simulink model "identyfikacja_zawor3_reczny"  (R2014b)
settings: Solver=ode5  StartTime=0.0  StopTime=41.25  FixedStep=0.05  RelTol=1e-3
values from neighbouring files (symbols this model uses):
  C3 = q/sqrt(H3pp)    [linearyzacja_analitycznie.m]    (also in wskaznikZawor3.m = parametry(1))
  R = 40    [charakterystyki_zawory_reczne.m]    (also in daneZawory_cz2.mat; nastawyLQ.m; pomiary.m; rhs.m)
  w = 5    [charakterystyka_pompa.m]    (also in charakterystyka_pompa_sterownik.m; dane14listopad.mat; danePompa.mat; pomiary.m)
  x03 = parametry(2)    [wskaznikZawor3.m]
settings Model: Creator=Michal  LastModifiedBy=Michal
settings DebuggingCC: UnderspecifiedInitializationDetection=Classic  MergeDetectMultiDrivingBlocksExec=none

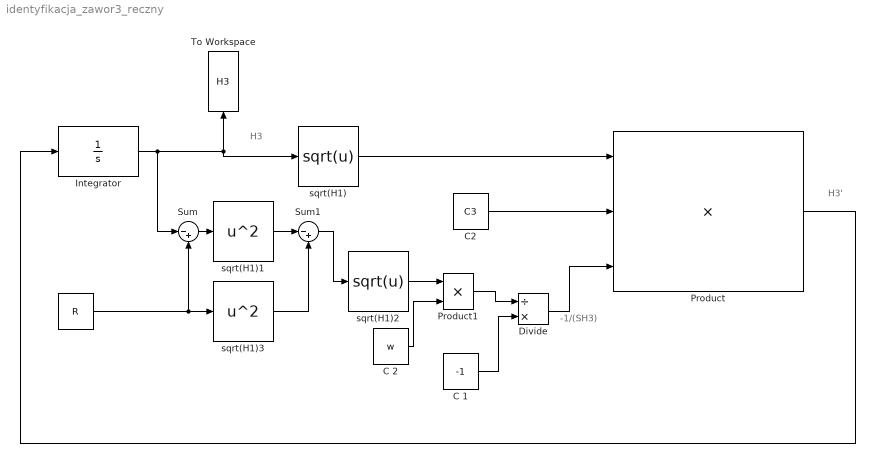
== system identyfikacja_zawor3_reczny ==
  note: -1/(SH3)
  note: H3'
  note: H3
  " " : Constant  Value=R
  C 1 : Constant  Value=-1
  C 2 : Constant  Value=w
  "C2 " : Constant  Value=C3
  Divide : Product  Inputs=/*
  Integrator : Integrator  InitialCondition=x03
  Product : Product  Inputs=3
  Product1 : Product
  Sum : Sum  Inputs=|-+
  Sum1 : Sum  Inputs=|-+
  To Workspace : ToWorkspace  VariableName=H3  SaveFormat=Structure With Time  SampleTime=-1
  sqrt(H1) : Fcn  Expr=sqrt(u)
  sqrt(H1)1 : Fcn  Expr=u^2
  sqrt(H1)2 : Fcn  Expr=sqrt(u)
  sqrt(H1)3 : Fcn  Expr=u^2
  wires:
  Integrator/1 -> To Workspace/1, sqrt(H1)/1, Sum/1
  Product/1 -> Integrator/1
  sqrt(H1)/1 -> Product/1
  "C2 "/1 -> Product/2
  " "/1 -> sqrt(H1)3/1, Sum/2
  Sum/1 -> sqrt(H1)1/1
  sqrt(H1)1/1 -> Sum1/1
  Sum1/1 -> sqrt(H1)2/1
  sqrt(H1)2/1 -> Product1/1
  C 2/1 -> Product1/2
  Product1/1 -> Divide/1
  Divide/1 -> Product/3
  sqrt(H1)3/1 -> Sum1/2
  C 1/1 -> Divide/2
